simulink library "V_Rep"  (R2015a)
settings: Solver=ode45  SolverMode=SingleTasking  StartTime=0.0  StopTime=10.0  RelTol=1e-3
undefined symbols (not defined in the file): T
libraries: aerolibanimutils x1
settings Model: CovMetricSettings=dwe  CovHtmlReporting=off  covSaveCumulativeToWorkspaceVar=off  CovSaveSingleToWorkspaceVar=off  CovModelRefEnable=off  CovExternalEMLEnable=on  Creator=laura  LastModifiedBy=HAROLD
settings DataIOCC: LimitDataPoints=off  SaveFormat=StructureWithTime
settings DebuggingCC: SFUnexpectedBacktrackingDiag=error  SFNoUnconditionalDefaultTransitionDiag=error
settings HardwareCC: ProdBitPerPointer=64  ProdLargestAtomicFloat=Float  ProdIntDivRoundTo=Zero  ProdEndianess=LittleEndian  ProdHWDeviceType=Specified
settings ModelReferenceCC: PropagateSignalLabelsOutOfModel=on
settings GRTTargetCC: TargetLangStandard=C99 (ISO)  GeneratePreprocessorConditionals=Use local settings

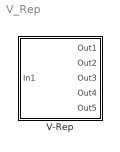
== system V_Rep ==
  V-Rep : Subsystem  mask(Bloque de V_Rep){Directory=Por Defecto, Parameter1=Péndulo de Furuta, Parameter2=T, Parameter3=3, Parameter6=on, Parameter7=4, Parameter8=C:\Program Files\V-REP3\V-REP_PRO_EDU}
      mask prompts: Directory "Directorio de V-Rep"; Parameter1 "Planta a emular"; Parameter2 "Tiempo de muestreo"; Parameter3 "sfdhg"; Parameter6 "Mostrar error de paso"; Parameter7 "Numero de salidas"; Parameter8 "dasads"
      mask help: Este bloque realiza una conexión con V_Rep, teniendo unas plantas ya preprogramadas para su mayor facilidad.
      mask init:
      | switch get_param(gcb,'Parameter1');
      |     case 'Péndulo de Furuta'
      |         t='3';
      |     case 'Bola Plato'
      |         t='1';
      |     case 'Bola Viga'
      |         t='2';
      |     case 'Otros'
      |         t='0';
      | end
      | set_param(gcb,'Parameter3',t);
      mask TypeOptions Directory: Por Defecto | C:\Program Files\V-REP3\V-REP_PRO_EDU
      mask Callback Directory:
      | DIR=get_param(gcb,'Directory');
      | 
      | if(strcmpi(DIR,'Por Defecto'));
      |     if ismac
      |         DIR='/Applications/V-REP_PRO_EDU_V3_6_2_Mac';
      |     elseif ispc
      |         DIR='C:\Program Files\V-REP3\V-REP_PRO_EDU'
      |     end
      | 
      | end
      | 
      | if ~strcmp(DIR,get_param(gcb,'Parameter8'))
      |     if ~exist(DIR, 'dir')
      |         baseException = MException('MYFUN:BadIndex','MYFUN:BadIndex');
      |         throw(baseException);
      |     else
      | 
      |         if~exist(strcat(DIR,'/credits.txt'), 'file')
      |            baseException = MException('MYFUN:BadIndex','V-Rep no está instalado en el directorio indicado');
      |            throw(baseException);
      |         else
      | 
      |             assignin('base','Path', {['-I' DIR '/programming/common/'],['-I' DIR '/programming/remoteApi/'],['-I' DIR '/programming/include/']});
      |             save('Path.mat','Path'),
      |             load('Path.mat');
      |             mex('-v',Path{1,1},Path{1,2},Path{1,3},'v.c','v_Rep_wrapper.c');
      |         end
      |     end
      |     set_param(gcb,'Parameter8',DIR)
      | end
      mask TypeOptions Parameter1: Péndulo de Furuta | Bola Plato | Bola Viga | Otros
      mask Callback Parameter1:
      | NM=str2num(get_param([gcb '/Demux2'],'Outputs'));
      | i = Simulink.Mask.get(gcb);
      | i=i.Parameters(6);
      | switch get_param(gcb,'Parameter1')
      |     case 'Péndulo de Furuta'
      |         i.set('Enabled','off');
      |         N=4;
      |     case 'Bola Plato'
      |         i.set('Enabled','off');
      |         N=4;
      |     case 'Bola Viga'
      |         i.set('Enabled','off');
      |         N=3;
      |     case 'Otros'
      |         i.set('Enabled','on');
      |         N=NM;
      | end
      | set_param(gcb,'Parameter7',num2str(N));
      | if N~=NM
      |     if getSimulinkBlockHandle([gcb '/Out' num2str(NM+1,'%01d')])~=-1 & strcmp(get_param(gcb,'Parameter6'),'on')
      |          delete_line(gcb,'Simulation Pace/1',['Out' num2str(NM+1,'%01d') '/1']);
      |          delete_block([gcb '/Out' num2str(NM+1,'%01d')]);
      |     end
      |     if N<NM
      |         for i=NM:-1:N+1
      |             delete_line(gcb,['Demux2/' num2str(i,'%01d')],['Out' num2str(i,'%01d') '/1']);
      |             delete_block([gcb '/Out' num2str(i,'%01d')]);
      |         end
      |                 set_param([gcb '/Demux2'],'Outputs',num2str(N))
      |     else
      |         set_param([gcb '/Demux2'],'Outputs',num2str(N))
      |         for i=NM+1:N
      |             add_block('simulink/Commonly Used Blocks/Out1',[gcb '/Out'  num2str(i,'%01d')]);
      |             add_line(gcb,['Demux2/' num2str(i,'%01d')],['Out' num2str(i,'%01d') '/1']);
      |         end
      |     end
      | 
      |     if getSimulinkBlockHandle([gcb '/Out' num2str(N+1,'%01d')]) ==-1 & strcmp(get_param(gcb,'Parameter6'),'on')
      |          add_block('simulink/Commonly Used Blocks/Out1',[gcb '/Out' num2str(N+1,'%01d')]);
      |          add_line(gcb,'Simulation Pace/1',['Out' num2str(N+1,'%01d') '/1']);
      |     end
      | 
      | end
      mask Callback Parameter6:
      | NM=get_param([gcb '/Demux2'],'Outputs');
      | if strcmp(get_param(gcb,'Parameter6'),'on')
      |     set_param([gcb '/Simulation Pace'],'OutputPaceError',get_param(gcb,'Parameter6'));
      |     if getSimulinkBlockHandle([gcb '/Out' NM+1]) ==-1
      |         add_block('simulink/Commonly Used Blocks/Out1',[gcb '/Out' NM+1]);
      |         add_line(gcb,'Simulation Pace/1',['Out' NM+1 '/1']);
      |     end
      | else
      |     if getSimulinkBlockHandle([gcb '/Out' NM+1])  ~=-1
      |         delete_line(gcb,'Simulation Pace/1',['Out' NM+1 '/1']);
      |         delete_block([gcb '/Out' NM+1]);
      |     end
      |     set_param([gcb '/Simulation Pace'],'OutputPaceError',get_param(gcb,'Parameter6'));
      | end
      mask Callback Parameter7:
      | NM=str2num(get_param([gcb '/Demux2'],'Outputs'));
      | N=str2num(get_param(gcb,'Parameter7'));
      | if N~=NM
      |     if getSimulinkBlockHandle([gcb '/Out' num2str(NM+1,'%01d')])~=-1 & strcmp(get_param(gcb,'Parameter6'),'on')
      |         delete_line(gcb,'Simulation Pace/1',['Out' num2str(NM+1,'%01d') '/1']);
      |         delete_block([gcb '/Out' num2str(NM+1,'%01d')]);
      |     end
      |     if N<NM
      |         for i=NM:-1:N+1
      |             delete_line(gcb,['Demux2/' num2str(i,'%01d')],['Out' num2str(i,'%01d') '/1']);
      |             delete_block([gcb '/Out' num2str(i,'%01d')]);
      |         end
      |     else
      |         set_param([gcb '/Demux2'],'Outputs',num2str(N))
      |         for i=NM+1:N
      |             add_block('simulink/Commonly Used Blocks/Out1',[gcb '/Out'  num2str(i,'%01d')]);
      |             add_line(gcb,['Demux2/' num2str(i,'%01d')],['Out' num2str(i,'%01d') '/1']);
      |         end
      |     end
      |     if getSimulinkBlockHandle([gcb '/Out' num2str(N+1,'%01d')]) ==-1 & strcmp(get_param(gcb,'Parameter6'),'on')
      |         add_block('simulink/Commonly Used Blocks/Out1',[gcb '/Out' num2str(N+1,'%01d')]);
      |         add_line(gcb,'Simulation Pace/1',['Out' num2str(N+1,'%01d') '/1']);
      |     end
      |     set_param([gcb '/Demux2'],'Outputs',num2str(N))
      | end
      mask DialogControl Control2 Prompt: Buscar
      mask DialogControl Control2 Callback:
      | path = uigetdir();
      | if path~=0
      | 
      |     p=Simulink.Mask.get(gcb)
      |     p.Parameters(1).TypeOptions={'Por Defecto',path};
      |     set_param(gcb,'Directory',1)
      |     if ~exist(path, 'dir')
      |         baseException = MException('V-Rep no está instalado en el directorio indicado','El directorio no existe');
      |         throw(baseException);
      |     else
      | 
      |         if~exist(strcat(path,'/credits.txt'), 'file')
      |            baseException = MException('MYFUN:BadIndex','V-Rep no está instalado en el directorio indicado');
      |            throw(baseException);
      |         else
      |             assignin('base','Path', {['-I' DIR '/programming/common/'],['-I' DIR '/programming/remoteApi/'],['-I' DIR '/programming/include/']});
      |             save('Path.mat','Path')
      |             load('Path.mat');
      |             mex('-v',Path{1,1},Path{1,2},Path{1,3},'v.c','v_Rep_wrapper.c');
      |         end
      |     end
      | end
      mask Display:
      | disp('V-Rep');
      | port_label('input', 1, 'u');
      | N= get_param(gcb,'Parameter7');
      | 
      | for i=1:str2num(N)
      |     port_label('output',i,['x' num2str(i)]);
      | end
      | if strcmp(get_param(gcb,'Parameter6'),'on')
      |     port_label('output',str2num(N)+1, 'Error');
      | end

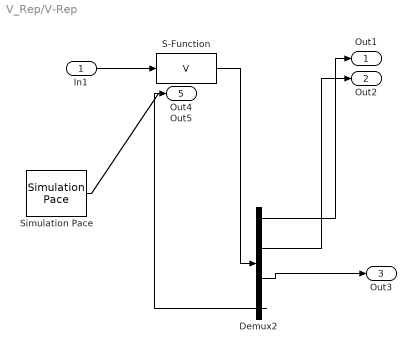
== system V_Rep/V-Rep ==
  In1 : Inport
  Demux2 : Demux
  S-Function : S-Function  FunctionName=V  Parameters=Parameter3,Parameter2,Parameter7  SFunctionModules=V_wrapper
  Simulation Pace : aerolibanimutils/Simulation Pace  SimulationPace=1  SleepMode=MATLAB Thread  OutputPaceError=on  SampleTime=Parameter2
  Out1 : Outport
  Out2 : Outport  Port=2
  Out3 : Outport  Port=3
  Out4 : Outport  Port=4
  Out5 : Outport  Port=5
  wires:
  Demux2/1 -> Out1/1
  S-Function/1 -> Demux2/1
  In1/1 -> S-Function/1
  Demux2/2 -> Out2/1
  Demux2/3 -> Out3/1
  Demux2/4 -> Out4/1
  Simulation Pace/1 -> Out5/1
